simulink model "talos_ekf"  (R2023a)
settings: Solver=FixedStepAuto  StartTime=0.0  StopTime=10  FixedStep=talosEkfCfg.sampleTime  RelTol=1e-3
undefined symbols (not defined in the file or in its folder): talosEkfCfg
libraries: sharedTrackingLibrary x1
settings Model: Creator=ethan  LastModifiedBy=ethan
settings OptimizationCC: DefaultParameterBehavior=Inlined  UseDivisionForNetSlopeComputation=on  GainParamInheritBuiltInType=on  UseFloatMulNetSlope=on  InlineInvariantSignals=on  PassReuseOutputArgsAs=Individual arguments  ZeroExternalMemoryAtStartup=off  ZeroInternalMemoryAtStartup=off  NoFixptDivByZeroProtection=on  EfficientFloat2IntCast=on  LifeSpan=1  OptimizeBlockOrder=speed  DifferentSizesBufferReuse=on  EfficientTunableParamExpr=on
settings DebuggingCC: ParameterTunabilityLossMsg=error
settings HardwareCC: ProdBitPerLong=64  ProdHWDeviceType=Intel->x86-64 (Linux 64)
settings SFSimCC: MATLABDynamicMemAlloc=off  SimTargetLang=C++
settings RTWCC: Description=Embedded Coder  SystemTargetFile=ert.tlc  GenCodeOnly=on  TemplateMakefile=ert_default_tmf  GenerateReport=on  IncludeHyperlinkInReport=on  TargetLang=C++  GenerateTraceInfo=on  GenerateTraceReport=on  GenerateTraceReportSl=on  GenerateTraceReportSf=on  GenerateTraceReportEml=on
settings CodeAppCC: ForceParamTrailComments=on  IgnoreCustomStorageClasses=off  OperatorAnnotations=on  SimulinkDataObjDesc=on  SFDataObjDesc=on  CustomSymbolStrGlobalVar=rt$N$M  CustomSymbolStrType=$N$M  CustomSymbolStrFcn=$N$M$F  CustomSymbolStrMacro=$N$M  InsertBlockDesc=on
settings ERTTargetCC: TargetLangStandard=C++11 (ISO)  GenerateSampleERTMain=on  IncludeMdlTerminateFcn=off  CombineSignalStateStructs=on  CodeInterfacePackaging=C++ class  SupportContinuousTime=on  SupportNonInlinedSFcns=on  SupportVariableSizeSignals=on  InlinedParameterPlacement=NonHierarchical  RootIOFormat=Structure reference  ERTCustomFileTemplate=example_file_process.tlc

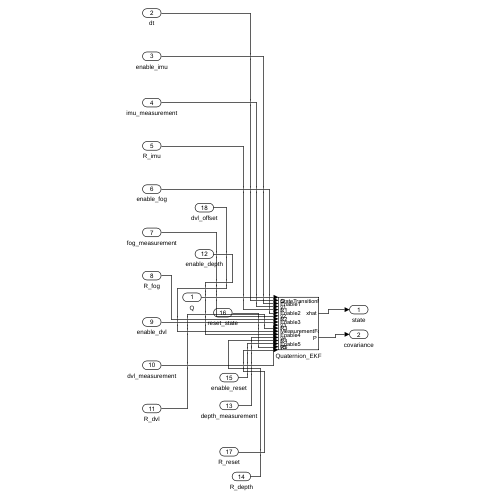
[thumbnail: Simulink's stored preview of the top-level diagram]
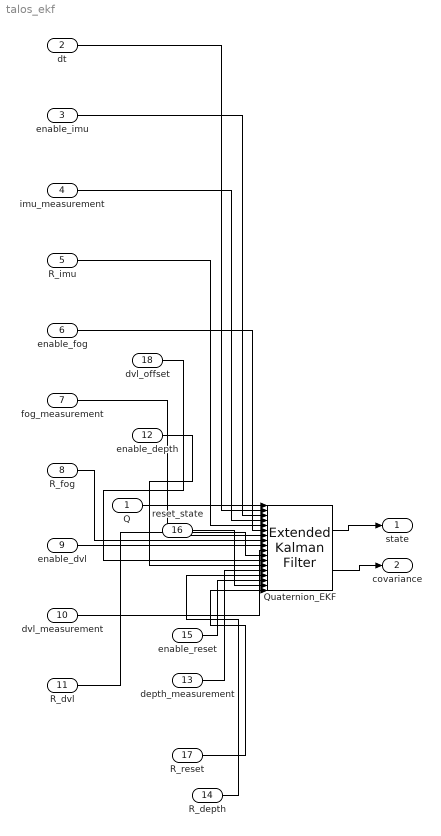
== system talos_ekf ==
  Q : Inport  OutDataTypeStr=double  PortDimensions=[16 16]
  dt : Inport  Port=2  OutDataTypeStr=double  PortDimensions=1
  enable_imu : Inport  Port=3  OutDataTypeStr=boolean  PortDimensions=1
  imu_measurement : Inport  Port=4  OutDataTypeStr=double  PortDimensions=8
  R_imu : Inport  Port=5  OutDataTypeStr=double  PortDimensions=[8 8]
  enable_fog : Inport  Port=6  OutDataTypeStr=boolean  PortDimensions=1
  fog_measurement : Inport  Port=7  OutDataTypeStr=double  PortDimensions=1
  R_fog : Inport  Port=8  OutDataTypeStr=double  PortDimensions=1
  enable_dvl : Inport  Port=9  OutDataTypeStr=boolean  PortDimensions=1
  dvl_measurement : Inport  Port=10  OutDataTypeStr=double  PortDimensions=3
  R_dvl : Inport  Port=11  OutDataTypeStr=double  PortDimensions=[3 3]
  enable_depth : Inport  Port=12  OutDataTypeStr=boolean  PortDimensions=1
  depth_measurement : Inport  Port=13  OutDataTypeStr=double  PortDimensions=1
  R_depth : Inport  Port=14  OutDataTypeStr=double  PortDimensions=1
  enable_reset : Inport  Port=15  OutDataTypeStr=boolean  PortDimensions=1
  reset_state : Inport  Port=16  OutDataTypeStr=double  PortDimensions=16
  R_reset : Inport  Port=17  OutDataTypeStr=double  PortDimensions=[16 16]
  dvl_offset : Inport  Port=18  PortDimensions=3
  Quaternion_EKF : sharedTrackingLibrary/Extended Kalman Filter  StateTransitionFcn=talos_state_transition  HasStateTransitionJacobianFcn=on  StateTransitionJacobianFcn=talos_state_jacobian  HasAdditiveProcessNoise=Additive  ProcessNoise=talosEkfCfg.processNoise  HasTimeVaryingProcessNoise=on  HasStateTransitionFcnExtraArgument=1  InitialState=talosEkfCfg.initialState  InitialStateCovariance=talosEkfCfg.initialCovariance  MeasurementFcn1=talos_measure_imu  HasMeasurementJacobianFcn1=on  MeasurementJacobianFcn1=talos_measure_imu_jacobian  HasMeasurementEnablePort1=on  HasAdditiveMeasurementNoise1=Additive  MeasurementNoise1=1  HasTimeVaryingMeasurementNoise1=on  HasMeasurementFcnExtraArgument1=0  HasMeasurementWrapping1=off  MeasurementFcn2=talos_measure_fog  HasMeasurementJacobianFcn2=on  MeasurementJacobianFcn2=talos_measure_fog_jacobian  HasMeasurementEnablePort2=on  HasAdditiveMeasurementNoise2=Additive  MeasurementNoise2=1  HasTimeVaryingMeasurementNoise2=on  HasMeasurementFcnExtraArgument2=0  HasMeasurementWrapping2=off  MeasurementFcn3=talos_measure_dvl  HasMeasurementJacobianFcn3=on  MeasurementJacobianFcn3=talos_measure_dvl_jacobian  HasMeasurementEnablePort3=on  HasAdditiveMeasurementNoise3=Additive  MeasurementNoise3=1  HasTimeVaryingMeasurementNoise3=on  HasMeasurementFcnExtraArgument3=1  HasMeasurementWrapping3=off  MeasurementFcn4=talos_measure_depth  HasMeasurementJacobianFcn4=on  MeasurementJacobianFcn4=talos_measure_depth_jacobian  HasMeasurementEnablePort4=on  HasAdditiveMeasurementNoise4=Additive  MeasurementNoise4=1  HasTimeVaryingMeasurementNoise4=on  HasMeasurementFcnExtraArgument4=0  HasMeasurementWrapping4=off  MeasurementFcn5=talos_measure_reset  HasMeasurementJacobianFcn5=on  MeasurementJacobianFcn5=talos_measure_reset_jacobian  HasMeasurementEnablePort5=on  HasAdditiveMeasurementNoise5=Additive  MeasurementNoise5=1  HasTimeVaryingMeasurementNoise5=on  HasMeasurementFcnExtraArgument5=0  HasMeasurementWrapping5=off  EnableMultirate=off  StateTransitionFcnSampleTime=1  MeasurementFcn1SampleTime=1  MeasurementFcn2SampleTime=1  MeasurementFcn3SampleTime=1  MeasurementFcn4SampleTime=1  MeasurementFcn5SampleTime=1  UseCurrentEstimator=on  OutputStateCovariance=on  DataType=double  SampleTime=talosEkfCfg.sampleTime  NumberOfMeasurements=5
  state : Outport  PortDimensions=16
  covariance : Outport  Port=2  PortDimensions=[16 16]
  wires:
  Q/1 -> Quaternion_EKF/1
  dt/1 -> Quaternion_EKF/2
  enable_imu/1 -> Quaternion_EKF/3
  imu_measurement/1 -> Quaternion_EKF/4
  R_imu/1 -> Quaternion_EKF/5
  enable_fog/1 -> Quaternion_EKF/6
  fog_measurement/1 -> Quaternion_EKF/7
  R_fog/1 -> Quaternion_EKF/8
  enable_dvl/1 -> Quaternion_EKF/9
  dvl_measurement/1 -> Quaternion_EKF/10
  R_dvl/1 -> Quaternion_EKF/11
  Quaternion_EKF/1 -> state/1
  Quaternion_EKF/2 -> covariance/1
  dvl_offset/1 -> Quaternion_EKF/12
  enable_depth/1 -> Quaternion_EKF/13
  depth_measurement/1 -> Quaternion_EKF/14
  R_depth/1 -> Quaternion_EKF/15
  enable_reset/1 -> Quaternion_EKF/16
  reset_state/1 -> Quaternion_EKF/17
  R_reset/1 -> Quaternion_EKF/18
